simulink model "Boeing787"  (R2013a)
settings: Solver=ode45  SolverMode=SingleTasking  StartTime=0.0  StopTime=10.0  RelTol=1e-3
values from neighbouring files (symbols this model uses):
  FuelBurn = [0 0 0 0 0 0 0 0 0 0 0 0 ... (18249 elements, 1x18249)]    [Benchmark_data1.mat]
undefined symbols (not defined in the file or in its folder): Gearbox_Torque
libraries: PowerFlowLib x27, simulink x5
(part 1 of 6)
settings Model: Creator=Bradford  LastModifiedBy=Andrew
settings DataIOCC: SignalLoggingSaveFormat=ModelDataLogs
settings OptimizationCC: BlockReduction=off  BooleanDataType=off
settings DebuggingCC: SaveWithParameterizedLinksMsg=none  SignalResolutionControl=TryResolveAllWithWarning  SolverPrmCheckMsg=none  MultiTaskDSMMsg=warning  MultiTaskCondExecSysMsg=none  StrictBusMsg=None
settings HardwareCC: TargetUnknown=on
settings RTWCC: IncludeERTFirstTime=on

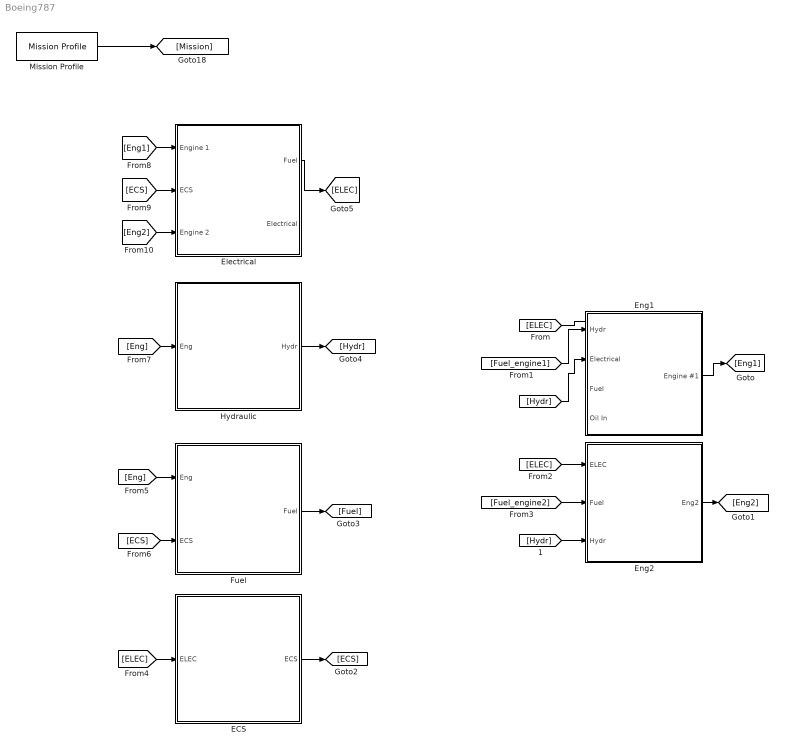
== system Boeing787 ==
  ECS : Subsystem
  Electrical : Subsystem
  Eng1 : Subsystem
  Eng2 : Subsystem
  Fuel : Subsystem
  Hydraulic : Subsystem
  Mission Profile : PowerFlowLib/Mission Profile/Mission Profile  mssn_check=off  mssn_prof=MSSN  del_P=0  del_T=0  del_rho=0  pres_msl=101.3  temp_msl=15  dens_msl=1.229
  wires:
  [ELEC] -> ?
  [Fuel_engine1] -> Eng1/1(Hydr)
  [Hydr] -> Eng1/2(Electrical)
  Eng1/1(Engine #1) -> [Eng1]
  [ELEC] -> Eng2/1(ELEC)
  [Fuel_engine2] -> Eng2/2(Fuel)
  [Hydr] -> Eng2/3(Hydr)
  Eng2/1(Eng2) -> [Eng2]
  [ELEC] -> ECS/1(ELEC)
  ECS/1(ECS) -> [ECS]
  [Eng] -> Fuel/1(Eng)
  [ECS] -> Fuel/2("ECS ")
  Fuel/1(Fuel) -> [Fuel]
  [Eng] -> Hydraulic/1(Eng)
  Hydraulic/1("Hydr ") -> [Hydr]
  [Eng1] -> Electrical/1(Engine 1)
  [ECS] -> Electrical/2("ECS ")
  Electrical/1(Fuel) -> [ELEC]
  Mission Profile/1 -> [Mission]
  [Eng2] -> Electrical/3(Engine 2)

== system Boeing787/ECS ==
  ELEC : Inport
  ECS : Outport
  wires:
  ELEC/1 -> ECS/1

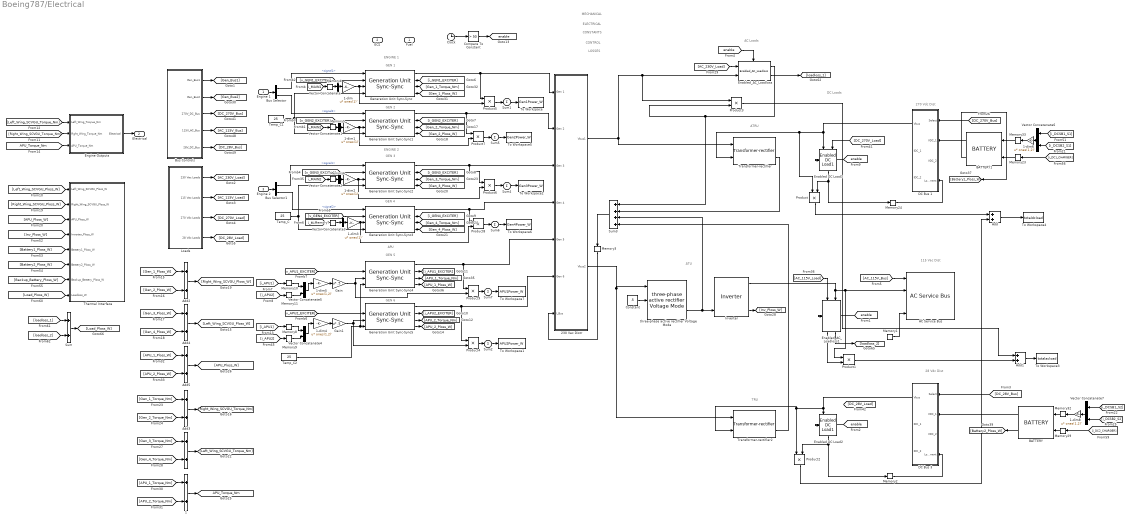
== system Boeing787/Electrical ==
  note: GEN 1
  note: ENGINE 1
  note: GEN 2
  note: GEN 3
  note: ENGINE 2
  note: GEN 4
  note: GEN 5
  note: APU
  note: GEN 6
  note: ATRU
  note: TRU
  note: ATU
  note: AC Loads
  note: 270 Vdc Dist
  note: 115 Vac Dist
  note: 28 Vdc Dist
  note: DC Loads
  note: CONSTANTS
  note: CONTROL
  note: LOSSES
  note: MECHANICAL
  note: ELECTRICAL
  Engine 1 : Inport
  "ECS " : Inport  Port=2
  Engine 2 : Inport  Port=3
  " " : Sum
  " 1" : Sum
  " Inverter" : PowerFlowLib/Energy & Power Systems/Electrical/Inverters/ Inverter  Trise=4e-6  Tfall=4e-6  fsw=2e3  Vcesat=1.2  Nofsw=6
  1-dim{,1..3} (4 alike) : Gain  Gain=ones(1)'  Multiplication=Matrix(u*K)
  1-dim{4..6,8} (4 alike) : Gain  Gain=ones(1,2)'  Multiplication=Matrix(u*K)
  230 Vac Distr : Subsystem
  AC Service Bus : PowerFlowLib/Energy & Power Systems/Electrical/Systems/AC Service Bus
  Add{,1..5} (6 alike) : Sum
  BATTERY : PowerFlowLib/Energy & Power Systems/Electrical/Battery/BATTERY  NO_CELLS=9  NO_MODULES=10  INITIAL_SOC=1
  BATTERY1 : PowerFlowLib/Energy & Power Systems/Electrical/Battery/BATTERY  NO_CELLS=9  NO_MODULES=10  INITIAL_SOC=1
  Bus Selector : BusSelector  OutputSignals=signal1,signal2
  Bus Selector1 : BusSelector  OutputSignals=signal1,signal2
  Bus Controls : Subsystem  mask{BUS1=Generator 1, BUS2=Generator 2, MBUS1=Generator Bus 1, ACTBUS1=Generator Bus 1, MBUS2=Generator Bus 2, ACTBUS2=Generator Bus 2, IDCBUS1=Battery 1, IDCBUS2=Battery 2}
      mask prompts: BUS1 "Source for Bus 1"; BUS2 "Source for Bus 2"; MBUS1 "Load on Main Bus 1 drawn from"; ACTBUS1 "Load on AC Transfer Bus 1 drawn from"; MBUS2 "Load on Main Bus 2 drawn from"; ACTBUS2 "Load on AC Transfer Bus 2 drawn from"; IDCBUS1 "Source for DC Service Bus 1"; IDCBUS2 "Source for DC Service Bus 2"
      mask help:
      | Specify the source from which different buses receive power. There are
      | 1. Two Generator buses (Bus 1-2)
      | 2. Two AC Main buses (Main Bus 1-2))
      | 3. Two AC Transfer buses and (AC Transfer Bus 1-2)
      | 4. Two DC Intermediate buses (DC Intermediate Bus 1-2)
      mask init:
      | switch BUS1
      |     case 1
      |         BUS1CONTROL = 1;
      |     case 2
      |         BUS1CONTROL = 2;
      |     case 3
      |         BUS1CONTROL = 3;
      |     case 4
      |         BUS1CONTROL = 4;
      | end
      | 
      | switch BUS2
      |     case 1
      |         BUS2CONTROL = 1;
      |     case 2
      |         BUS2CONTROL = 2;
      |     case 3
      |         BUS2CONTROL = 3;
      |     case 4
      |         BUS2CONTROL = 4;
      | end
      | 
      | switch MBUS1
      |     case 1
      |         MBUS1CONTROL = 1;
      |     case 2
      |         MBUS1CONTROL = 2;
      | end
      | 
      | switch ACTBUS1
      |     case 1
      |         ACTBUS1CONTROL = 1;
      |     case 2
      |         ACTBUS1CONTROL = 2;
      | end
      | 
      | switch MBUS2
      |     case 1
      |         MBUS2CONTROL = 1;
      |     case 2
      |         MBUS2CONTROL = 2;
      | end
      | 
      | switch ACTBUS2
      |     case 1
      |         ACTBUS2CONTROL = 1;
      |     case 2
      |         ACTBUS2CONTROL = 2;
      | end
      | 
      | switch IDCBUS1
      |     case 1
      |         IDCBUS1CONTROL = 1;
      |     case 2
      |         IDCBUS1CONTROL = 2;
      | end
      | 
      | switch IDCBUS2
      |     case 1
      |         IDCBUS2CONTROL = 1;
      |     case 2
      |         IDCBUS2CONTROL = 2;
      | end
      mask TypeOptions BUS1: Generator 1  | APU  | GND | AUX SUPPLY
      mask TypeOptions BUS2: Generator 2  | APU  | GND | AUX SUPPLY
      mask TypeOptions MBUS1: Generator Bus 1 | Generator Bus 2
      mask TypeOptions ACTBUS1: Generator Bus 1 | Generator Bus 2
      mask TypeOptions MBUS2: Generator Bus 1 | Generator Bus 2
      mask TypeOptions ACTBUS2: Generator Bus 1 | Generator Bus 2
      mask TypeOptions IDCBUS1: Battery 1 | Battery 2
      mask TypeOptions IDCBUS2: Battery 1 | Battery 2
  Clock : Clock
  Compare To Constant : simulink/Logic and Bit Operations/Compare To Constant  relop=>  const=50  OutDataTypeStr=uint8
  Constant : Constant  Value=.5
  DC Bus 1 : Subsystem  mask(DC Service Bus){}
      mask help: Service Bus
  DC Bus 3 : Subsystem  mask(DC Service Bus){}
      mask help: Service Bus
  Enabled DC Load1 : PowerFlowLib/Energy & Power Systems/Electrical/Loads/Enabled  DC Load1
  Enabled DC Load2 : PowerFlowLib/Energy & Power Systems/Electrical/Loads/Enabled  DC Load1
  Enabled_AC_Loadloss : PowerFlowLib/Energy & Power Systems/Electrical/Loads/Enabled_AC_Loadloss  P=500  PF=0.85  ILRMS=0  R=10000  X=10000
  Enabled_AC_Loadloss1 : PowerFlowLib/Energy & Power Systems/Electrical/Loads/Enabled_AC_Loadloss  P=500  PF=0.85  ILRMS=0  R=10000  X=10000
  Engine Outputs : Subsystem
  Gain : Gain  Gain=.5  Multiplication=Matrix(u*K)
  Gain1 : Gain  Gain=.5  Multiplication=Matrix(u*K)
  Generation Unit Sync-Sync{,1..5} (6 alike) : PowerFlowLib/Energy & Power Systems/Electrical/Systems/Generation Unit Sync-Sync  machine_mode=100kVA_Gen  Rs=0.0163  Xls=0.00054  Xmd=0.66176  Xmq=0.00099  R_fd=0.016  Xlfd=0.2092  R_1d=0.2047  Xl1d=0.6524  R_1q=0.0429  R_2q=0.0429  Xl1q=0.0639  Xl2q=0.0639  ws=377  RTL=0.001  XTL=0.1  KA=20  KF=0.063  T_f=0.35  TA=0.2  KE=1  TE=0.314  SB=100000  VBDQ=100  wB=377  P=6  H=0.1777  R_conv_gen=0.05  mc_gen=10000  Vnom=115  fan_load='init_fan_characteristics.mat'  exciter_param='exciter.mat'
  Loads : Subsystem
  Memory{1..11,23..24,29,32..33} (16 alike) : Memory
  Product{,1..9} (10 alike) : Product
  Sum : Sum
  Sum{1..2,4..7} (6 alike) : Sum  Inputs=+
  Sum3 : Sum  Inputs=++++
  Temp_C : Constant  Value=25
  Temp_C1 : Constant  Value=25
  Temp_C2 : Constant  Value=25
  Thermal Interface : Subsystem
  To Workspace : ToWorkspace  VariableName=Gen1Power_W  SampleTime=10  SaveFormat=Structure With Time
  To Workspace1 : ToWorkspace  VariableName=APU2Power_W  SampleTime=10  SaveFormat=Structure With Time
  To Workspace2 : ToWorkspace  VariableName=Gen3Power_W  SampleTime=10  SaveFormat=Structure With Time
  To Workspace3 : ToWorkspace  VariableName=totalacload  SampleTime=-1  SaveFormat=Timeseries
  To Workspace4 : ToWorkspace  VariableName=totaldcload  SampleTime=-1  SaveFormat=Timeseries
  To Workspace5 : ToWorkspace  VariableName=Gen2Power_W  SampleTime=10  SaveFormat=Structure With Time
  To Workspace6 : ToWorkspace  VariableName=Gen4Power_W  SampleTime=10  SaveFormat=Structure With Time
  To Workspace7 : ToWorkspace  VariableName=APU1Power_W  SampleTime=10  SaveFormat=Structure With Time
  Transformer-rectifier : PowerFlowLib/Energy & Power Systems/Electrical/Systems/Transformer-rectifier  pu=1
  Transformer-rectifier2 : PowerFlowLib/Energy & Power Systems/Electrical/Systems/Transformer-rectifier  pu=1
  Vector Concatenate{,1..3} (4 alike) : Concatenate  NumInputs=1  Mode=Multidimensional array  ConcatenateDimension=2
  Vector Concatenate{4..7} (4 alike) : Concatenate  Mode=Multidimensional array  ConcatenateDimension=2
  three-phase active rectifier Voltage Mode : PowerFlowLib/Energy & Power Systems/Electrical/Rectifiers/three-phase  active rectifier Voltage Mode  L=1e-3  C=1e-4
  Fuel : Outport
  Electrical : Outport  Port=2
  tag scope: APU_Torque_Nm=global, enable=global
  wires:
  Generation Unit Sync-Sync/1 -> Product5/1, 230 Vac Distr/1(Gen 1)
  Generation Unit Sync-Sync1/1 -> Product7/1, 230 Vac Distr/2(Gen 2)
  Generation Unit Sync-Sync2/1 -> Product6/1, 230 Vac Distr/3(Gen 3)
  Generation Unit Sync-Sync3/1 -> Product8/1, 230 Vac Distr/4(Gen 4)
  Generation Unit Sync-Sync4/1 -> Product9/1, 230 Vac Distr/5(Gen 5)
  Generation Unit Sync-Sync5/1 -> Product4/1, 230 Vac Distr/6(Gen 6)
  Engine 1/1 -> Bus Selector/1
  230 Vac Distr/1(Vbus1) -> Product3/1, Enabled_AC_Loadloss/2, Transformer-rectifier/1
  230 Vac Distr/2(Vbus2) -> three-phase active rectifier Voltage Mode/1, Transformer-rectifier2/1
  [enable] -> Enabled_AC_Loadloss/Enable
  DC Bus 1/1(Vbus) -> Enabled DC Load1/1, Product/1, Transformer-rectifier/2
  DC Bus 3/1(Vbus) -> Product2/1, Transformer-rectifier2/2, Enabled DC Load2/1
  Enabled DC Load1/1 -> Product/2, Memory24/1
  Memory24/1 -> DC Bus 1/4(Load current)
  Enabled DC Load2/1 -> Product2/2, Memory2/1
  Memory2/1 -> DC Bus 3/4(Load current)
  [enable] -> Enabled DC Load1/Enable
  [enable] -> Enabled_AC_Loadloss1/Enable
  [enable] -> Enabled DC Load2/Enable
  Transformer-rectifier2/2 -> Sum3/4
  Transformer-rectifier/2 -> Sum3/2
  Enabled_AC_Loadloss/1 -> Product3/2, Sum3/1
  Sum3/1 -> Memory3/1
  Memory3/1 -> 230 Vac Distr/7(I_Bus)
  Memory1/1 -> AC Service Bus/4
  " Inverter"/1 -> Product1/1, AC Service Bus/2, Enabled_AC_Loadloss1/2
  BATTERY/1 -> DC Bus 3/2(VDC_1)
  BATTERY1/1 -> DC Bus 1/2(VDC_1)
  Enabled_AC_Loadloss1/1 -> Product1/2
  Product/1 -> Add/1
  Memory32/1 -> BATTERY/1
  1-dim8/1 -> Memory32/1
  [i_DCSB1_S2] -> Vector Concatenate7/1
  [i_DCSB2_S2] -> Vector Concatenate7/2
  Vector Concatenate7/1 -> 1-dim8/1
  Memory29/1 -> BATTERY/2
  [i_DC2_CHARGER] -> Memory29/1
  Memory33/1 -> BATTERY1/1
  Memory23/1 -> BATTERY1/2
  1-dim6/1 -> Memory33/1
  [i_DCSB1_S1] -> Vector Concatenate6/1
  [i_DCSB2_S1] -> Vector Concatenate6/2
  Vector Concatenate6/1 -> 1-dim6/1
  [i_DC1_CHARGER] -> Memory23/1
  [AC_230V_Load] -> Enabled_AC_Loadloss/1
  Enabled_AC_Loadloss/2 -> [loadloss_1]
  Product2/1 -> Add/2
  Add/1 -> To Workspace4/1
  Add1/1 -> To Workspace3/1
  Product1/1 -> Add1/2
  Product3/1 -> Add1/1
  Enabled_AC_Loadloss1/2 -> [loadloss_2]
  [AC_115V_Load] -> Enabled_AC_Loadloss1/1
  [DC_270V_Load] -> Enabled DC Load1/2
  Loads/1(230 Vac Loads) -> [AC_230V_Load]
  Loads/2(115 Vac Loads) -> [AC_115V_Load]
  Loads/3(270 Vdc Loads) -> [DC_270V_Load]
  Loads/4(28 Vdc Loads) -> [DC_28V_Load]
  [DC_270V_Bus] -> DC Bus 1/1(Select)
  [DC_28V_Bus] -> DC Bus 3/1(Select)
  [AC_115V_Bus] -> AC Service Bus/1
  Bus Controls/1(Gen_Bus1) -> [Gen_Bus1]
  Bus Controls/2(Gen_Bus2) -> [Gen_Bus2]
  Bus Controls/5(28V_DC_Bus) -> [DC_28V_Bus]
  BATTERY/2 -> [Battery2_Ploss_W]
  BATTERY1/2 -> [Battery1_Ploss_W]
  Bus Controls/4(115V_AC_Bus) -> [AC_115V_Bus]
  Bus Controls/3(270V_DC_Bus) -> [DC_270V_Bus]
  [i_MAIN1] -> Memory4/1
  [i_MAIN2] -> Memory6/1
  [i_MAIN2] -> Memory7/1
  [i_MAIN1] -> Memory5/1
  Memory7/1 -> Vector Concatenate3/1
  Vector Concatenate3/1 -> 1-dim3/1
  1-dim3/1 -> Product8/2, Generation Unit Sync-Sync3/3
  Memory6/1 -> Vector Concatenate2/1
  Vector Concatenate2/1 -> 1-dim2/1
  1-dim2/1 -> Product6/2, Generation Unit Sync-Sync2/3
  Memory5/1 -> Vector Concatenate1/1
  Vector Concatenate1/1 -> 1-dim1/1
  1-dim1/1 -> Product7/2, Generation Unit Sync-Sync1/3
  Memory4/1 -> Vector Concatenate/1
  Vector Concatenate/1 -> 1-dim/1
  1-dim/1 -> Product5/2, Generation Unit Sync-Sync/3
  Clock/1 -> Compare To Constant/1
  Compare To Constant/1 -> [enable]
  Bus Selector/1 -> Generation Unit Sync-Sync/1  "<signal1>"
  Bus Selector/2 -> Generation Unit Sync-Sync1/1  "<signal2>"
  Engine 2/1 -> Bus Selector1/1
  Bus Selector1/1 -> Generation Unit Sync-Sync2/1  "<signal1>"
  Bus Selector1/2 -> Generation Unit Sync-Sync3/1  "<signal2>"
  [v_GEN1_EXCITER] -> Generation Unit Sync-Sync/2
  Generation Unit Sync-Sync/2 -> [i_GEN1_EXCITER]
  Generation Unit Sync-Sync1/2 -> [i_GEN2_EXCITER]
  Generation Unit Sync-Sync2/2 -> [i_GEN3_EXCITER]
  Generation Unit Sync-Sync3/2 -> [i_GEN4_EXCITER]
  [v_GEN2_EXCITER] -> Generation Unit Sync-Sync1/2
  [v_GEN3_EXCITER] -> Generation Unit Sync-Sync2/2
  [v_GEN4_EXCITER] -> Generation Unit Sync-Sync3/2
  Temp_C1/1 -> Generation Unit Sync-Sync1/4, Generation Unit Sync-Sync/4
  Temp_C/1 -> Generation Unit Sync-Sync3/4, Generation Unit Sync-Sync2/4
  Product4/1 -> Sum2/1
  Sum2/1 -> To Workspace1/1
  Vector Concatenate4/1 -> 1-dim4/1
  [i_APU2] -> Memory9/1
  [i_APU1] -> Memory8/1
  Memory8/1 -> Vector Concatenate4/1
  Memory9/1 -> Vector Concatenate4/2
  [v_APU2_EXCITER] -> Generation Unit Sync-Sync5/2
  Temp_C2/1 -> Generation Unit Sync-Sync4/4, Generation Unit Sync-Sync5/4
  Vector Concatenate5/1 -> 1-dim5/1
  [i_APU2] -> Memory11/1
  [i_APU1] -> Memory10/1
  Memory10/1 -> Vector Concatenate5/1
  Memory11/1 -> Vector Concatenate5/2
  [v_APU1_EXCITER] -> Generation Unit Sync-Sync4/2
  Product5/1 -> Sum1/1
  Sum1/1 -> To Workspace/1
  Product6/1 -> Sum4/1
  Sum4/1 -> To Workspace2/1
  Product7/1 -> Sum5/1
  Sum5/1 -> To Workspace5/1
  Product8/1 -> Sum6/1
  Sum6/1 -> To Workspace6/1
  Product9/1 -> Sum7/1
  Sum7/1 -> To Workspace7/1
  Engine Outputs/1(Electrical) -> Electrical/1
  [Left_Wing_SCVGU_Torque_Nm] -> Engine Outputs/1(Left_Wing_Toqrue_Nm)
  [Right_Wing_SCVGU_Torque_Nm] -> Engine Outputs/2(Rght_Wing_Torque_Nm)
  [APU_Torque_Nm] -> Engine Outputs/3(APU_Torque_Nm)
  [Left_Wing_SCVGU_Ploss_W] -> Thermal Interface/1(Left_Wing_SCVGU_Ploss_W)
  [Right_Wing_SCVGU_Ploss_W] -> Thermal Interface/2(Right_Wing_SCVGU_Ploss_W)
  [APU_Ploss_W] -> Thermal Interface/3(APU_Ploss_W)
  [Inv_Ploss_W] -> Thermal Interface/4(Inverter_Ploss_W)
  [Battery1_Ploss_W] -> Thermal Interface/5(Battery1_Ploss_W)
  [Battery2_Ploss_W] -> Thermal Interface/6(Battery2_Ploss_W)
  [Backup_Battery_Ploss_W] -> Thermal Interface/7(Backup_Battery_Ploss_W)
  [Load_Ploss_W] -> Thermal Interface/8(Loadloss_W)
  [loadloss_1] -> Sum/1
  [loadloss_2] -> Sum/2
  Sum/1 -> [Load_Ploss_W]
  Generation Unit Sync-Sync4/3 -> [APU_1_Torque_Nm]
  Generation Unit Sync-Sync5/3 -> [APU_2_Torque_Nm]
  Generation Unit Sync-Sync4/2 -> [i_APU1_EXCITER]
  Generation Unit Sync-Sync4/4 -> [APU_1_Ploss_W]
  Generation Unit Sync-Sync5/4 -> [APU_2_Ploss_W]
  Generation Unit Sync-Sync5/2 -> [i_APU2_EXCITER]
  Generation Unit Sync-Sync/4 -> [Gen_1_Ploss_W]
  Generation Unit Sync-Sync/3 -> [Gen_1_Torque_Nm]
  three-phase active rectifier Voltage Mode/2 -> Sum3/3, " Inverter"/3
  Generation Unit Sync-Sync1/3 -> [Gen_2_Torque_Nm]
  Generation Unit Sync-Sync1/4 -> [Gen_2_Ploss_W]
  Add4/1 -> [Left_Wing_SCVGU_Ploss_W]
  Add2/1 -> [Right_Wing_SCVGU_Ploss_W]
  [Gen_1_Ploss_W] -> Add2/1
  [Gen_2_Ploss_W] -> Add2/2
  Generation Unit Sync-Sync3/4 -> [Gen_4_Ploss_W]
  Generation Unit Sync-Sync2/4 -> [Gen_3_Ploss_W]
  [Gen_4_Ploss_W] -> Add4/2
  [Gen_3_Ploss_W] -> Add4/1
  Add3/1 -> [Right_Wing_SCVGU_Torque_Nm]
  " "/1 -> [Left_Wing_SCVGU_Torque_Nm]
  Generation Unit Sync-Sync3/3 -> [Gen_4_Torque_Nm]
  Generation Unit Sync-Sync2/3 -> [Gen_3_Torque_Nm]
  [Gen_1_Torque_Nm] -> Add3/1
  [Gen_2_Torque_Nm] -> Add3/2
  [Gen_3_Torque_Nm] -> " "/1
  [Gen_4_Torque_Nm] -> " "/2
  1-dim5/1 -> Gain/1
  Gain/1 -> Product9/2, Generation Unit Sync-Sync4/3
  Gain1/1 -> Product4/2, Generation Unit Sync-Sync5/3
  1-dim4/1 -> Gain1/1
  " 1"/1 -> [APU_Torque_Nm]
  [APU_1_Torque_Nm] -> " 1"/1
  [APU_2_Torque_Nm] -> " 1"/2
  Add5/1 -> [APU_Ploss_W]
  [APU_2_Ploss_W] -> Add5/2
  [APU_1_Ploss_W] -> Add5/1
  Constant/1 -> three-phase active rectifier Voltage Mode/2
  " Inverter"/3 -> [Inv_Ploss_W]
